simulink model "Factorial_using_for_loop"  (R2021a)
settings: Solver=FixedStepDiscrete  StartTime=0.0  StopTime=1  RelTol=1e-3  EnableMultiTasking=on
settings Model: Creator=Karim  LastModifiedBy=Karim
settings DataIOCC: ReturnWorkspaceOutputs=off
settings OptimizationCC: DefaultParameterBehavior=Inlined  InlineInvariantSignals=on  EnableMemcpy=off  LifeSpan=1  EfficientTunableParamExpr=on
settings DebuggingCC: UnderspecifiedInitializationDetection=Classic  MergeDetectMultiDrivingBlocksExec=none  SFMachineParentedDataDiag=warning  ArithmeticOperatorsInVariantConditions=warning
settings ModelReferenceCC: PropagateSignalLabelsOutOfModel=off
settings SFSimCC: MATLABDynamicMemAlloc=off  CustomCodeUndefinedFunction=UseInterfaceOnly
settings RTWCC: SystemTargetFile=ert.tlc  GenCodeOnly=on  TemplateMakefile=ert_default_tmf  GenerateReport=on  IncludeHyperlinkInReport=on  LaunchReport=on  GenerateTraceInfo=on  GenerateTraceReport=on  GenerateTraceReportSl=on  GenerateTraceReportSf=on  GenerateTraceReportEml=on
settings CodeAppCC: ForceParamTrailComments=on  IgnoreCustomStorageClasses=off  OperatorAnnotations=on  SimulinkDataObjDesc=on  SFDataObjDesc=on  MATLABFcnDesc=on  InsertBlockDesc=on  StateflowObjectComments=on  MATLABSourceComments=on
settings ERTTargetCC: MultiwordLength=2048  GenerateSampleERTMain=on  InlinedParameterPlacement=NonHierarchical  ERTCustomFileTemplate=example_file_process.tlc

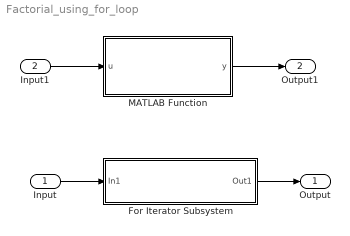
== system Factorial_using_for_loop ==
  Input : Inport
  Input1 : Inport  Port=2
  For Iterator Subsystem : Subsystem  TreatAsAtomicUnit=on
  MATLAB Function : MATLAB Function  TreatAsAtomicUnit=on
  Output : Outport
  Output1 : Outport  Port=2
  wires:
  Input1/1 -> MATLAB Function/1(u)
  MATLAB Function/1(y) -> Output1/1
  Input/1 -> For Iterator Subsystem/1(In1)
  For Iterator Subsystem/1(Out1) -> Output/1

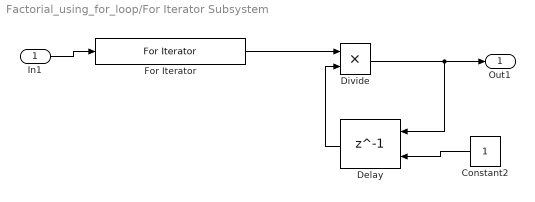
== system Factorial_using_for_loop/For Iterator Subsystem ==
  In1 : Inport
  Constant2 : Constant
  Delay : Delay  DelayLength=1  InitialConditionSource=Input port
      settings: InputPortMap=u0,p4
  Divide : Product  Inputs=**
  For Iterator : ForIterator  IterationSource=external
  Out1 : Outport
  wires:
  For Iterator/1 -> Divide/1
  Constant2/1 -> Delay/2
  Divide/1 -> Delay/1, Out1/1
  Delay/1 -> Divide/2
  In1/1 -> For Iterator/1

== matlab function Factorial_using_for_loop/MATLAB Function ==
  data: u input; y output
function y = factorial_function(u)
    fact = 1;
    while u > 0
        fact = fact * u;
        u = u - 1;
    end
    y = fact;
end
